simulink model "Model"  (R2019b)
settings: Solver=FixedStepAuto  StartTime=0.0  StopTime=100  FixedStep=1e-5  RelTol=1e-3
PostLoadFcn:
  | Kp = 1;
  | Ki = 3;
  | Kd = 0;
  | 
  | Kawu = 1; % default value
libraries: simulink x1
settings Model: Creator=Szczepi
settings DataIOCC: ReturnWorkspaceOutputs=off
settings DebuggingCC: ArithmeticOperatorsInVariantConditions=warning
settings SFSimCC: SimUseLocalCustomCode=off  CustomCodeUndefinedFunction=UseInterfaceOnly
settings RTWCC: RTWUseLocalCustomCode=off
settings ConfigComp: CovBoundaryAbsTol=1.0e-5

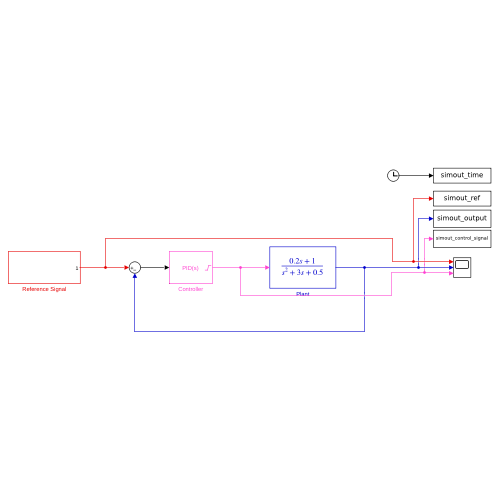
[thumbnail: Simulink's stored preview of the top-level diagram]
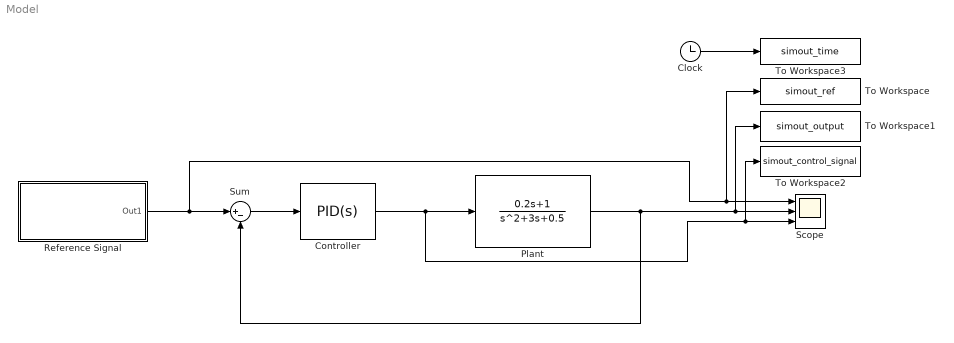
== system Model ==
  Clock : Clock
  Controller : simulink/Continuous/PID Controller  Controller=PID  Form=Parallel  TimeDomain=Continuous-time  SampleTime=-1  IntegratorMethod=Forward Euler  FilterMethod=Forward Euler  ControllerParametersSource=internal  P=Kp  I=Ki  D=Kd  N=100  UseFilter=on  TunerSelectOption=Transfer Function Based (PID Tuner App)  InitialConditionSource=internal  InitialConditionForIntegrator=0  InitialConditionForFilter=0  DifferentiatorICPrevScaledInput=0  ExternalReset=none  TrackingMode=off  Kt=1  LimitOutput=on  UpperSaturationLimit=10  LowerSaturationLimit=-10  LinearizeAsGain=on  AntiWindupMode=back-calculation  Kb=Kawu  POutMin=[]  POutMax=[]  IOutMin=[]  IOutMax=[]  DOutMin=[]  DOutMax=[]  NOutMin=[]  NOutMax=[]  SumOutMin=[]  SumOutMax=[]  SaturationOutMin=[]  SaturationOutMax=[]  PParamMin=[]  PParamMax=[]  IParamMin=[]  IParamMax=[]  DParamMin=[]  DParamMax=[]  NParamMin=[]  NParamMax=[]  KbParamMin=[]  KbParamMax=[]  KtParamMin=[]  KtParamMax=[]  KbOutMin=[]  KbOutMax=[]  KtOutMin=[]  KtOutMax=[]  IntegratorOutMin=[]  IntegratorOutMax=[]  FilterOutMin=[]  FilterOutMax=[]  SumI1OutMin=[]  SumI1OutMax=[]  SumI2OutMin=[]  SumI2OutMax=[]  SumI3OutMin=[]  SumI3OutMax=[]  SumI4OutMin=[]  SumI4OutMax=[]  SumDOutMin=[]  SumDOutMax=[]  DifferentiatorOutMin=[]  DifferentiatorOutMax=[]  FilterDiffOutCoefMin=[]  FilterDiffOutCoefMax=[]  ReciprocalOutMin=[]  ReciprocalOutMax=[]  SumDenOutMin=[]  SumDenOutMax=[]  SumNumOutMin=[]  SumNumOutMax=[]  DivideOutMin=[]  DivideOutMax=[]  IntegratorContinuousStateAttributes=''  IntegratorStateMustResolveToSignalObject=off  IntegratorRTWStateStorageClass=Auto  FilterContinuousStateAttributes=''  FilterStateMustResolveToSignalObject=off  FilterRTWStateStorageClass=Auto  ParallelPVariant=InternalParameters  IdealPVariant=Disabled  IVariant=InternalParameters  DVariant=InternalParameters  IntegratorVariant=Continuous  SatVariant=Enabled  AWVariant=BackCalculation  PCopyVariant=Disabled  TRVariant=Disabled  FdbkBlocksVariant=Forward  IdealPFdbkVariant=Disabled  SatFdbkVariant=Disabled  DerivativeFilterVariant=ContFilter  NVariant=InternalParameters  NCopyVariant=Disabled  FilterICVariant=InternalICsFilter  IntegratorICVariant=InternalICs  ExternalResetVariant=Disabled  TRSumVariant=Passthrough  SumFdbkVariant=Disabled  SumVariant=Sum_PID
  Plant : TransferFcn  Numerator=[0.2 1]  Denominator=[1 3 0.5]
  Reference Signal : Subsystem
  Scope : Scope  NumInputPorts=3
  Sum : Sum  Inputs=|+-
  To Workspace : ToWorkspace  VariableName=simout_ref  SampleTime=-1
  To Workspace1 : ToWorkspace  VariableName=simout_output  SampleTime=-1
  To Workspace2 : ToWorkspace  VariableName=simout_control_signal  SampleTime=-1
  To Workspace3 : ToWorkspace  VariableName=simout_time  SampleTime=-1
  wires:
  Plant/1 -> Sum/2, To Workspace1/1, Scope/2
  Sum/1 -> Controller/1
  Reference Signal/1(Out1) -> To Workspace/1, Scope/1, Sum/1
  Controller/1 -> To Workspace2/1, Scope/3, Plant/1
  Clock/1 -> To Workspace3/1

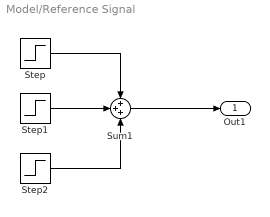
== system Model/Reference Signal ==
  Step : Step  After=10  SampleTime=0
  Step1 : Step  Time=50  After=-15  SampleTime=0
  Step2 : Step  Time=55  After=10  SampleTime=0
  Sum1 : Sum  Inputs=+++
  Out1 : Outport  VectorParamsAs1DForOutWhenUnconnected=off
  wires:
  Step2/1 -> Sum1/3
  Step/1 -> Sum1/1
  Sum1/1 -> Out1/1
  Step1/1 -> Sum1/2
